simulink model "analise"  (R2018a)
settings: Solver=ode1  StartTime=0.0  StopTime=Tsimu  FixedStep=h  RelTol=1e-3
values from neighbouring files (symbols this model uses):
  A = [(rgo*Cwro2 - Cwpg2) (rgo*Cwro3 - Cwpg3); (Cwro2 - Cwpo2) (Cwro3 - Cwpo3)]    [init.m]
  a0 = r0    (= 458.312763766)    [init.m]
  B = [1 0]'    [init.m]
  C = g/Aw*[1 1]    [init.m]
  f0 = 1/1000    (= 0.001)    [init.m]
  h = 1    [init.m]
  K0 = place(A, B, [-1 -0.002])    [init.m]
  N0 = 1/(C*inv(-1*(A - B*K0))*B)    [init.m]
  r0 = (rgo*Cwro4 - Cwpg4) - (rgo*Cwro3 - Cwpg3)*(Cwro4 - Cwpo4)/(Cwro3 - Cwpo3)    (= 458.312763766)    [init.m]
  Tsimu = 100e3    (= 100000)    [init.m]
  x0 = [-12 4]'    [init.m]
settings Model: Creator=Raposo  LastModifiedBy=raposo
settings OptimizationCC: LifeSpan=inf
settings DebuggingCC: AllowSymbolicDim=off  SFExecutionAtInitializationDiag=none
settings HardwareCC: ProdBitPerSizeT=32  ProdBitPerPtrDiffT=32  ProdWordSize=32  ProdHWDeviceType=Specified
settings CodeAppCC: StateflowObjectComments=on

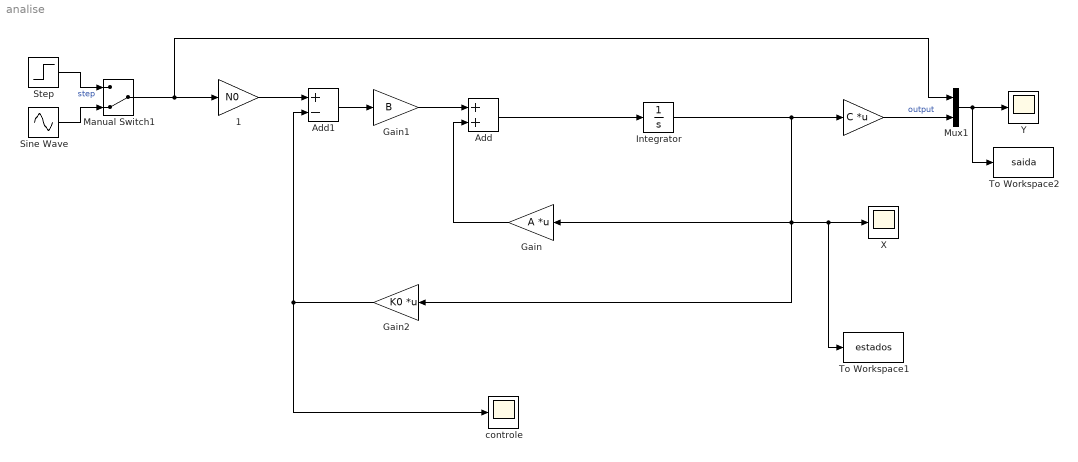
== system analise ==
  " " : Gain  Gain=C  Multiplication=Matrix(K*u)
  " 1" : Gain  Gain=N0
  Add : Sum
  Add1 : Sum  Inputs=+-
  Gain : Gain  Gain=A  Multiplication=Matrix(K*u)
  Gain1 : Gain  Gain=B
  Gain2 : Gain  Gain=K0  Multiplication=Matrix(K*u)
  Integrator : Integrator  InitialCondition=x0
  Manual Switch1 : ManualSwitch  CurrentSetting=0
  Mux1 : Mux  Inputs=2
  Sine Wave : Sin  Amplitude=a0  Frequency=f0  SampleTime=0
  Step : Step  Time=Tsimu/2  After=r0  SampleTime=h
  To Workspace1 : ToWorkspace  VariableName=estados  SampleTime=-1
  To Workspace2 : ToWorkspace  VariableName=saida  SampleTime=-1
  X : Scope
  Y : Scope
  controle : Scope
  wires:
  Mux1/1 -> Y/1, To Workspace2/1
  " "/1 -> Mux1/2  "output"
  Add1/1 -> Gain1/1
  Add/1 -> Integrator/1
  Integrator/1 -> " "/1, Gain2/1, To Workspace1/1, X/1, Gain/1
  Gain2/1 -> controle/1, Add1/2
  " 1"/1 -> Add1/1
  Step/1 -> Manual Switch1/1  "step"
  Sine Wave/1 -> Manual Switch1/2
  Manual Switch1/1 -> Mux1/1, " 1"/1
  Gain1/1 -> Add/1
  Gain/1 -> Add/2
